simulink model "sumulacionTpBolitaaa"  (R2019b)
settings: Solver=ode4  StartTime=0.0  StopTime=5  FixedStep=10e-6  RelTol=1e-3
undefined symbols (not defined in the file or in its folder): A0, Acd, B0, Bcd, c, C0, Ccd, Dcd, DiscIntNeverNeededParam, K, L, Pade, Tsample, u0, x0, x0f
libraries: cstblocks x2
settings Model: Creator=mpier  LastModifiedBy=rochi
settings ConfigComp: PLC_TargetIDE=codesys23

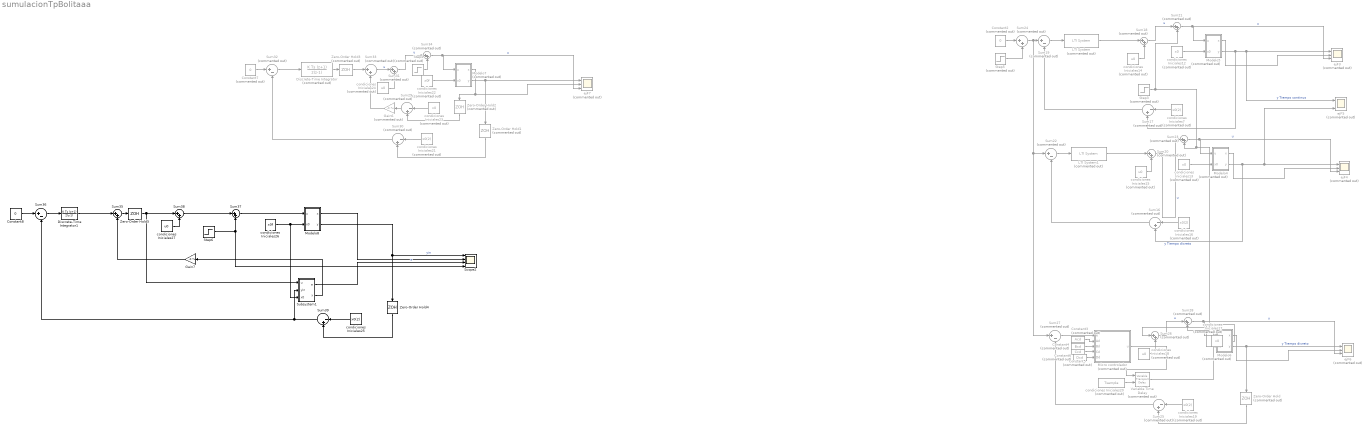
== system sumulacionTpBolitaaa ==
  " Micro controlador" : MATLAB Function  Commented=on  TreatAsAtomicUnit=on  SystemSampleTime=Tsample
  Constant2 : Constant  Commented=on  Value=0
  Constant3 : Constant  Commented=on  Value=Acd
  Constant4 : Constant  Commented=on  Value=Bcd
  Constant5 : Constant  Commented=on  Value=Ccd
  Constant6 : Constant  Commented=on  Value=Dcd
  Constant7 : Constant  Commented=on  Value=0
  Constant8 : Constant  Value=0
  Discrete-Time Integrator : DiscreteIntegrator  Commented=on  IntegratorMethod=Integration: Trapezoidal  gainval=Ki  SampleTime=Tsample  ICPrevOutput=DiscIntNeverNeededParam  ICPrevScaledInput=DiscIntNeverNeededParam
  Discrete-Time Integrator1 : DiscreteIntegrator  IntegratorMethod=Integration: Trapezoidal  gainval=Ki  SampleTime=Tsample  ICPrevOutput=DiscIntNeverNeededParam  ICPrevScaledInput=DiscIntNeverNeededParam
  Gain6 : Gain  Commented=on  Gain=-K  Multiplication=Matrix(K*u)
  Gain7 : Gain  Gain=-K  Multiplication=Matrix(K*u)
  LTI System : cstblocks/LTI System  Commented=on  sys=c*Pade  IC=[]
  LTI System1 : cstblocks/LTI System  Commented=on  sys=Cd  IC=[]
  Modelo4 : Subsystem  Commented=on
  Modelo5 : Subsystem  Commented=on
  Modelo6 : Subsystem  Commented=on
  Modelo7 : Subsystem  Commented=on
  Modelo8 : Subsystem
  Scope2 : Scope  NumInputPorts=4
  Step3 : Step  Commented=on  Time=2.5  After=100e-3  SampleTime=0
  Step4 : Step  Commented=on  Time=2.5  After=10  SampleTime=0
  Step5 : Step  Commented=on  After=1e-3  SampleTime=0
  Step6 : Step  Time=2.5  After=1e-3  SampleTime=0
  Subsystem1 : Subsystem
  Sum{16..17,25,29..30} (5 alike) : Sum  Commented=on  Inputs=|-+  OutDataTypeStr=double
  Sum{18,20..21,23,26,28,31,34} (8 alike) : Sum  Commented=on  Inputs=|++
  Sum{19,22,27,32} (4 alike) : Sum  Commented=on  Inputs=|+-  OutDataTypeStr=double
  Sum24 : Sum  Commented=on  Inputs=|++  OutDataTypeStr=double
  Sum33 : Sum  Commented=on  Inputs=|++  OutDataTypeStr=double
  Sum35 : Sum  Inputs=|++
  Sum36 : Sum  Inputs=|+-  OutDataTypeStr=double
  Sum37 : Sum  Inputs=|++
  Sum38 : Sum  Inputs=|++
  Sum39 : Sum  Inputs=|-+  OutDataTypeStr=double
  Variable Time Delay : VariableTransportDelay  Commented=on  MaximumDelay=10
  Zero-Order Hold : ZeroOrderHold  Commented=on  SampleTime=Tsample
  Zero-Order Hold1 : ZeroOrderHold  Commented=on  SampleTime=-1
  Zero-Order Hold2 : ZeroOrderHold  Commented=on  SampleTime=-1
  Zero-Order Hold3 : ZeroOrderHold  Commented=on  SampleTime=-1
  Zero-Order Hold4 : ZeroOrderHold  SampleTime=-1
  Zero-Order Hold5 : ZeroOrderHold  SampleTime=-1
  condiciones Iniciales{12..13,17,23} (4 alike) : Constant  Commented=on  Value=x0
  condiciones Iniciales{14..15,18,24} (4 alike) : Constant  Commented=on  Value=u0
  condiciones Iniciales{7,16,19,21} (4 alike) : Constant  Commented=on  Value=x0(2)
  condiciones Iniciales20 : Constant  Commented=on  Value=Tsample
  condiciones Iniciales22 : Constant  Commented=on  Value=x0f
  condiciones Iniciales25 : Constant  Value=x0(2)
  condiciones Iniciales26 : Constant  Value=x0f
  condiciones Iniciales27 : Constant  Value=u0
  ejF{3..4,6..7} (4 alike) : Scope  Commented=on  NumInputPorts=3
  ejF5 : Scope  Commented=on  NumInputPorts=2
  wires:
  condiciones Iniciales14/1 -> Sum18/2
  Modelo5/2(y) -> ejF5/1, ejF3/1, Sum17/2  "y Tiempo continuo"
  Sum19/1 -> LTI System/1
  Sum18/1 -> Sum21/1  "u"
  Sum17/1 -> Sum19/2
  Modelo5/1(x) -> ejF3/2
  Sum21/1 -> ejF3/3, Modelo5/1(u)  "u"
  condiciones Iniciales7/1 -> Sum17/1
  condiciones Iniciales12/1 -> Modelo5/2(x0)
  LTI System/1 -> Sum18/1
  condiciones Iniciales16/1 -> Sum16/1
  Sum23/1 -> ejF4/3, Modelo4/1(u)  "u"
  Sum16/1 -> Sum22/2
  Sum20/1 -> Sum23/1  "u"
  Modelo4/1(x) -> ejF4/2
  Sum22/1 -> LTI System1/1
  condiciones Iniciales15/1 -> Sum20/2
  Modelo4/2(y) -> ejF5/2, ejF4/1, Sum16/2  "y Tiempo dicreto"
  condiciones Iniciales13/1 -> Modelo4/2(x0)
  LTI System1/1 -> Sum20/1
  Constant2/1 -> Sum24/1
  Step5/1 -> Sum24/2
  Step3/1 -> Sum28/2, Sum23/2, Sum21/2
  condiciones Iniciales19/1 -> Sum25/1
  condiciones Iniciales18/1 -> Sum26/2
  Sum27/1 -> " Micro controlador"/1(e)
  Sum24/1 -> Sum19/1, Sum27/1, Sum22/1
  Sum28/1 -> ejF6/3, Modelo6/1(u)  "u"
  Sum26/1 -> Sum28/1  "u"
  Modelo6/1(x) -> ejF6/2
  condiciones Iniciales17/1 -> Modelo6/2(x0)
  Modelo6/2(y) -> ejF6/1, Zero-Order Hold/1  "y Tiempo dicreto"
  Sum25/1 -> Sum27/2
  Constant3/1 -> " Micro controlador"/2(Ad)
  Constant4/1 -> " Micro controlador"/3(Bd)
  Constant5/1 -> " Micro controlador"/4(Cd)
  Constant6/1 -> " Micro controlador"/5(Dd)
  " Micro controlador"/1(u) -> Variable Time Delay/1
  Variable Time Delay/1 -> Sum26/1
  condiciones Iniciales20/1 -> Variable Time Delay/2
  Zero-Order Hold/1 -> Sum25/2
  Modelo7/1(x) -> ejF7/2, Zero-Order Hold2/1
  Sum33/1 -> Sum31/1  "u"
  condiciones Iniciales23/1 -> Sum29/1
  Sum31/1 -> Sum34/1  "u"
  Modelo7/2(y) -> ejF7/1, Zero-Order Hold1/1
  Gain6/1 -> Sum33/2
  Sum32/1 -> Discrete-Time Integrator/1
  Step4/1 -> Sum34/2
  Discrete-Time Integrator/1 -> Zero-Order Hold3/1
  Sum34/1 -> ejF7/3, Modelo7/1(u)  "u"
  condiciones Iniciales21/1 -> Sum30/1
  Sum30/1 -> Sum32/2
  Sum29/1 -> Gain6/1
  condiciones Iniciales24/1 -> Sum31/2
  condiciones Iniciales22/1 -> Modelo7/2(x0)
  Constant7/1 -> Sum32/1
  Zero-Order Hold1/1 -> Sum30/2
  Zero-Order Hold2/1 -> Sum29/2
  Zero-Order Hold3/1 -> Sum33/1
  Sum36/1 -> Discrete-Time Integrator1/1
  Modelo8/2(y) -> Zero-Order Hold4/1, Scope2/1  "yin"
  Sum37/1 -> Modelo8/1(u)
  Modelo8/1(x) -> Scope2/2
  Sum35/1 -> Zero-Order Hold5/1
  condiciones Iniciales25/1 -> Sum39/1
  Sum38/1 -> Sum37/1
  Subsystem1/2(x) -> Gain7/1
  condiciones Iniciales27/1 -> Sum38/2
  condiciones Iniciales26/1 -> Subsystem1/3(x0), Modelo8/2(x0)
  Gain7/1 -> Sum35/2
  Discrete-Time Integrator1/1 -> Sum35/1
  Subsystem1/1(e) -> Scope2/3  "e"
  Sum39/1 -> Sum36/2, Subsystem1/2(yin)
  Zero-Order Hold4/1 -> Sum39/2
  Zero-Order Hold5/1 -> Subsystem1/1(u), Sum38/1
  Constant8/1 -> Sum36/1
  Step6/1 -> Sum37/2, Scope2/4

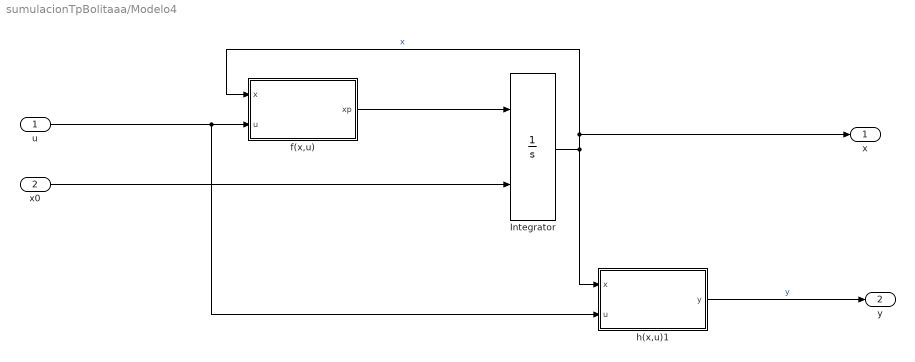
== system sumulacionTpBolitaaa/Modelo4 ==
  u : Inport
  x0 : Inport  Port=2
  Integrator : Integrator  InitialConditionSource=external
  f(x,u) : MATLAB Function  TreatAsAtomicUnit=on
  h(x,u)1 : MATLAB Function  TreatAsAtomicUnit=on
  x : Outport
  y : Outport  Port=2
  wires:
  Integrator/1 -> x/1, f(x,u)/1(x), h(x,u)1/1(x)  "x"
  f(x,u)/1(xp) -> Integrator/1
  x0/1 -> Integrator/2
  u/1 -> h(x,u)1/2(u), f(x,u)/2(u)
  h(x,u)1/1(y) -> y/1  "y"

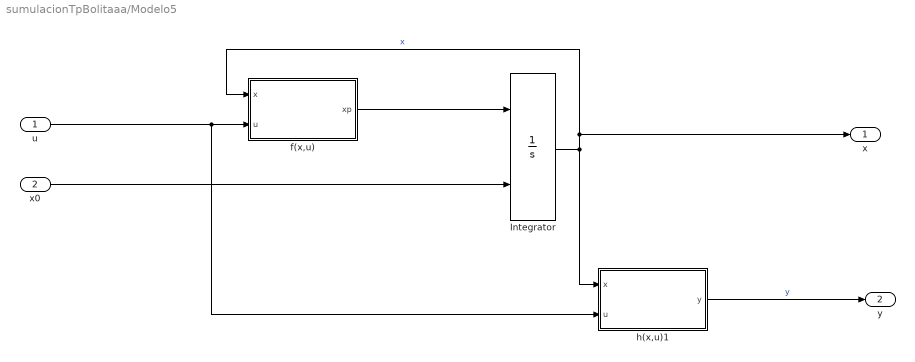
== system sumulacionTpBolitaaa/Modelo5 ==
  u : Inport
  x0 : Inport  Port=2
  Integrator : Integrator  InitialConditionSource=external
  f(x,u) : MATLAB Function  TreatAsAtomicUnit=on
  h(x,u)1 : MATLAB Function  TreatAsAtomicUnit=on
  x : Outport
  y : Outport  Port=2
  wires:
  Integrator/1 -> x/1, f(x,u)/1(x), h(x,u)1/1(x)  "x"
  f(x,u)/1(xp) -> Integrator/1
  x0/1 -> Integrator/2
  u/1 -> h(x,u)1/2(u), f(x,u)/2(u)
  h(x,u)1/1(y) -> y/1  "y"

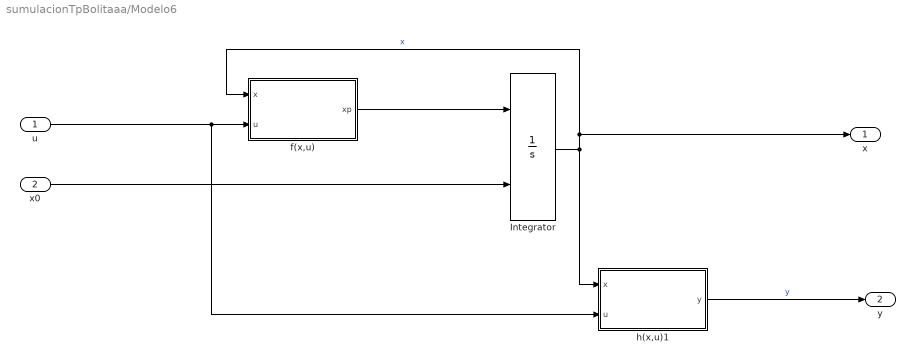
== system sumulacionTpBolitaaa/Modelo6 ==
  u : Inport
  x0 : Inport  Port=2
  Integrator : Integrator  InitialConditionSource=external
  f(x,u) : MATLAB Function  TreatAsAtomicUnit=on
  h(x,u)1 : MATLAB Function  TreatAsAtomicUnit=on
  x : Outport
  y : Outport  Port=2
  wires:
  Integrator/1 -> x/1, f(x,u)/1(x), h(x,u)1/1(x)  "x"
  f(x,u)/1(xp) -> Integrator/1
  x0/1 -> Integrator/2
  u/1 -> h(x,u)1/2(u), f(x,u)/2(u)
  h(x,u)1/1(y) -> y/1  "y"

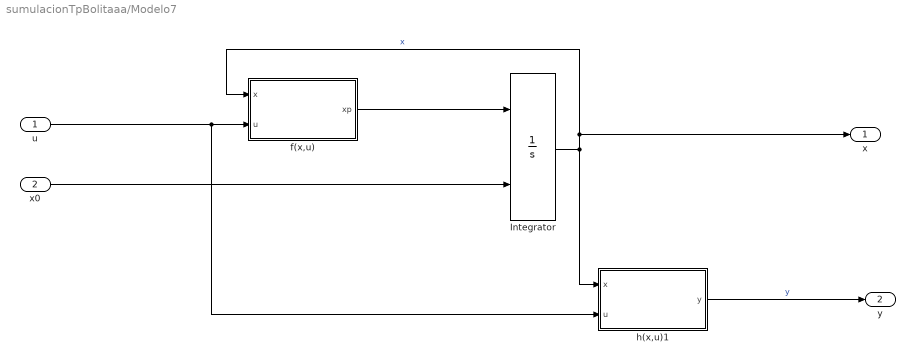
== system sumulacionTpBolitaaa/Modelo7 ==
  u : Inport
  x0 : Inport  Port=2
  Integrator : Integrator  InitialConditionSource=external
  f(x,u) : MATLAB Function  TreatAsAtomicUnit=on
  h(x,u)1 : MATLAB Function  TreatAsAtomicUnit=on
  x : Outport
  y : Outport  Port=2
  wires:
  Integrator/1 -> x/1, f(x,u)/1(x), h(x,u)1/1(x)  "x"
  f(x,u)/1(xp) -> Integrator/1
  x0/1 -> Integrator/2
  u/1 -> h(x,u)1/2(u), f(x,u)/2(u)
  h(x,u)1/1(y) -> y/1  "y"

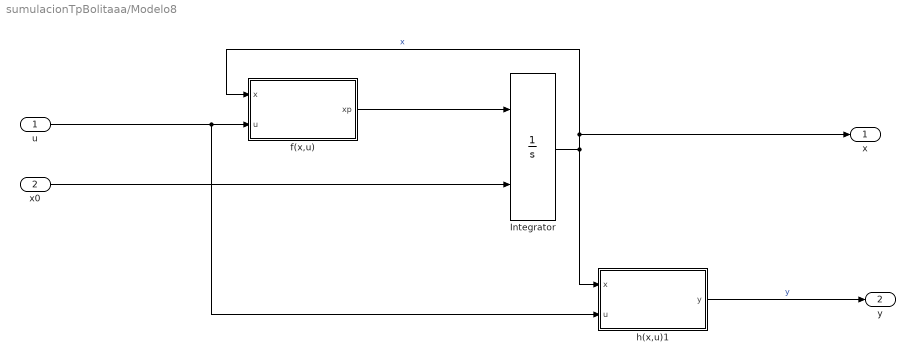
== system sumulacionTpBolitaaa/Modelo8 ==
  u : Inport
  x0 : Inport  Port=2
  Integrator : Integrator  InitialConditionSource=external
  f(x,u) : MATLAB Function  TreatAsAtomicUnit=on
  h(x,u)1 : MATLAB Function  TreatAsAtomicUnit=on
  x : Outport
  y : Outport  Port=2
  wires:
  Integrator/1 -> x/1, f(x,u)/1(x), h(x,u)1/1(x)  "x"
  f(x,u)/1(xp) -> Integrator/1
  x0/1 -> Integrator/2
  u/1 -> h(x,u)1/2(u), f(x,u)/2(u)
  h(x,u)1/1(y) -> y/1  "y"

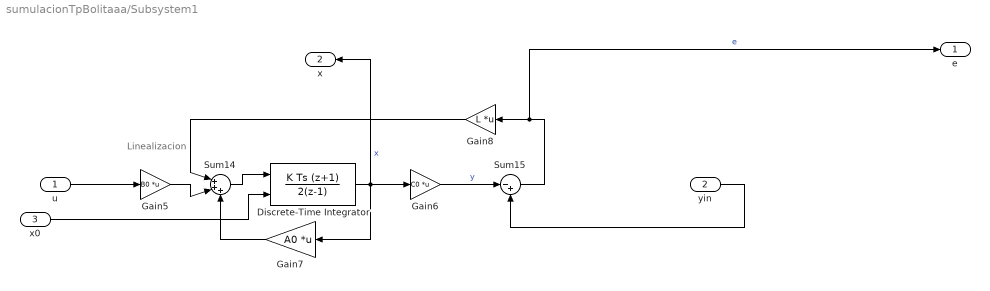
== system sumulacionTpBolitaaa/Subsystem1 ==
  note: Linealizacion
  u : Inport
  yin : Inport  Port=2
  x0 : Inport  Port=3
  Discrete-Time Integrator : DiscreteIntegrator  IntegratorMethod=Integration: Trapezoidal  InitialConditionSource=external  SampleTime=Tsample  ICPrevOutput=DiscIntNeverNeededParam  ICPrevScaledInput=DiscIntNeverNeededParam
  Gain5 : Gain  Gain=B0  Multiplication=Matrix(K*u)
  Gain6 : Gain  Gain=C0  Multiplication=Matrix(K*u)
  Gain7 : Gain  Gain=A0  Multiplication=Matrix(K*u)
  Gain8 : Gain  Gain=L  Multiplication=Matrix(K*u)
  Sum14 : Sum  Inputs=|+++
  Sum15 : Sum  Inputs=|-+
  e : Outport
  x : Outport  Port=2
  wires:
  u/1 -> Gain5/1
  Sum14/1 -> Discrete-Time Integrator/1
  yin/1 -> Sum15/2
  Discrete-Time Integrator/1 -> x/1, Gain7/1, Gain6/1  "x"
  Gain7/1 -> Sum14/3
  Sum15/1 -> e/1, Gain8/1  "e"
  Gain6/1 -> Sum15/1  "y"
  Gain5/1 -> Sum14/2
  Gain8/1 -> Sum14/1
  x0/1 -> Discrete-Time Integrator/2

== matlab function sumulacionTpBolitaaa/Modelo4/f(x,u) ==
  data: x input; u input; xp output
function xp = f(x,u)



R=4;%resistencia del inductor
 L=1;%inductancia del electro iman
 m=0.2;%masa de la bolita
 g=10;%aceleracion de la grabedad
 

ids=(-(x(1)^2)/(L/R))+(u/L);

F1s=(0.5*((2+x(1))^2))/((1-x(2))^2);
F2s=(0.5*((2-x(1))^2))/((1+x(2))^2);
vds=-g+(F1s/m)-(F2s/m);

xp=[ids;x(3);vds];

== matlab function sumulacionTpBolitaaa/Modelo4/h(x,u)1 ==
  data: x input; u input; y output
function y = h(x,u)



y=x(2);

== matlab function sumulacionTpBolitaaa/Modelo5/f(x,u) ==
  data: x input; u input; xp output
function xp = f(x,u)



R=4;%resistencia del inductor
 L=1;%inductancia del electro iman
 m=0.2;%masa de la bolita
 g=10;%aceleracion de la grabedad
 

ids=(-(x(1)^2)/(L/R))+(u/L);

F1s=(0.5*((2+x(1))^2))/((1-x(2))^2);
F2s=(0.5*((2-x(1))^2))/((1+x(2))^2);
vds=-g+(F1s/m)-(F2s/m);

xp=[ids;x(3);vds];

== matlab function sumulacionTpBolitaaa/Modelo5/h(x,u)1 ==
  data: x input; u input; y output
function y = h(x,u)



y=x(2);

== matlab function sumulacionTpBolitaaa/ Micro controlador ==
  data: e input; u output; Ad input; Bd input; Cd input; Dd input
function u = fcn(e,Ad,Bd,Cd,Dd)

persistent xp;

if isempty(xp)
    xp =[0;0;0;0];
end
xp1=[0;0;0;0];
xp1=Ad*xp+Bd*e;
u=transpose(Cd)*xp+Dd*e;

xp=xp1;
end

== matlab function sumulacionTpBolitaaa/Modelo6/f(x,u) ==
  data: x input; u input; xp output
function xp = f(x,u)



R=4;%resistencia del inductor
 L=1;%inductancia del electro iman
 m=0.2;%masa de la bolita
 g=10;%aceleracion de la grabedad
 

ids=(-(x(1)^2)/(L/R))+(u/L);

F1s=(0.5*((2+x(1))^2))/((1-x(2))^2);
F2s=(0.5*((2-x(1))^2))/((1+x(2))^2);
vds=-g+(F1s/m)-(F2s/m);

xp=[ids;x(3);vds];

== matlab function sumulacionTpBolitaaa/Modelo6/h(x,u)1 ==
  data: x input; u input; y output
function y = h(x,u)



y=x(2);

== matlab function sumulacionTpBolitaaa/Modelo7/f(x,u) ==
  data: x input; u input; xp output
function xp = f(x,u)



R=4;%resistencia del inductor
 L=1;%inductancia del electro iman
 m=0.2;%masa de la bolita
 g=10;%aceleracion de la grabedad
 

ids=(-(x(1)^2)/(L/R))+(u/L);

F1s=(0.5*((2+x(1))^2))/((1-x(2))^2);
F2s=(0.5*((2-x(1))^2))/((1+x(2))^2);
vds=-g+(F1s/m)-(F2s/m);

xp=[ids;x(3);vds];

== matlab function sumulacionTpBolitaaa/Modelo7/h(x,u)1 ==
  data: x input; u input; y output
function y = h(x,u)



y=x(2);

== matlab function sumulacionTpBolitaaa/Modelo8/f(x,u) ==
  data: x input; u input; xp output
function xp = f(x,u)



R=4;%resistencia del inductor
 L=1;%inductancia del electro iman
 m=0.2;%masa de la bolita
 g=10;%aceleracion de la grabedad
 

ids=(-(x(1)^2)/(L/R))+(u/L);

F1s=(0.5*((2+x(1))^2))/((1-x(2))^2);
F2s=(0.5*((2-x(1))^2))/((1+x(2))^2);
vds=-g+(F1s/m)-(F2s/m);

xp=[ids;x(3);vds];

== matlab function sumulacionTpBolitaaa/Modelo8/h(x,u)1 ==
  data: x input; u input; y output
function y = h(x,u)



y=x(2);
